simulink model "Estimator_Model_T_variable"  (R2017b)
settings: Solver=FixedStepAuto  StartTime=0.0  StopTime=T  FixedStep=0.01  RelTol=1e-3
values from neighbouring files (symbols this model uses):
  c = 0.02    [mainscript.m]
  Cf = 80000    [Init_for_washout_filter.m]
  Cr = 85000    [Init_for_washout_filter.m]
  L = lf+lr    (= 2.55)    [Init_for_washout_filter.m]
  lf = 0.41*2.55    (= 1.0455)    [Init_for_washout_filter.m]
  lr = 2.55-lf    (= 1.5045)    [Init_for_washout_filter.m]
  m = 3    [mainscript.m]
  mass = 1435-80    (= 1355)    [Init_for_washout_filter.m]
  rollGrad = 5*(pi/180)    (= 0.0872664625997)    [Init_for_washout_filter.m]
  rx = 0.4    [Init_for_washout_filter.m]
  T_w = 1    [mainscript.m]
  Tau = 0.3    [mainscript.m]
settings Model: Creator=gandh  LastModifiedBy=gandh

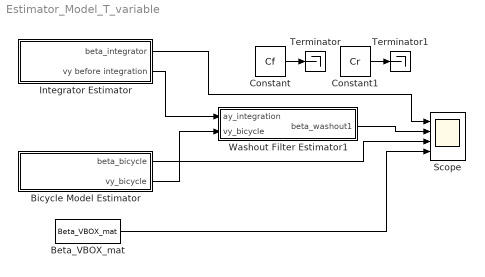
== system Estimator_Model_T_variable ==
  Beta_VBOX_mat : FromWorkspace  VariableName=Beta_VBOX_mat  SampleTime=0
  Bicycle Model Estimator : Subsystem
  Constant : Constant  Value=Cf
  Constant1 : Constant  Value=Cr
  Integrator Estimator : Subsystem
  Scope : Scope  NumInputPorts=4
  Terminator : Terminator
  Terminator1 : Terminator
  Washout Filter Estimator1 : Subsystem
  wires:
  Integrator Estimator/1(beta_integrator) -> Scope/1
  Bicycle Model Estimator/2(vy_bicycle) -> Washout Filter Estimator1/2(vy_bicycle)
  Beta_VBOX_mat/1 -> Scope/4
  Bicycle Model Estimator/1(beta_bicycle) -> Scope/3
  Constant/1 -> Terminator/1
  Constant1/1 -> Terminator1/1
  Integrator Estimator/2(vy before integration) -> Washout Filter Estimator1/1(ay_integration)
  Washout Filter Estimator1/1(beta_washout1) -> Scope/2

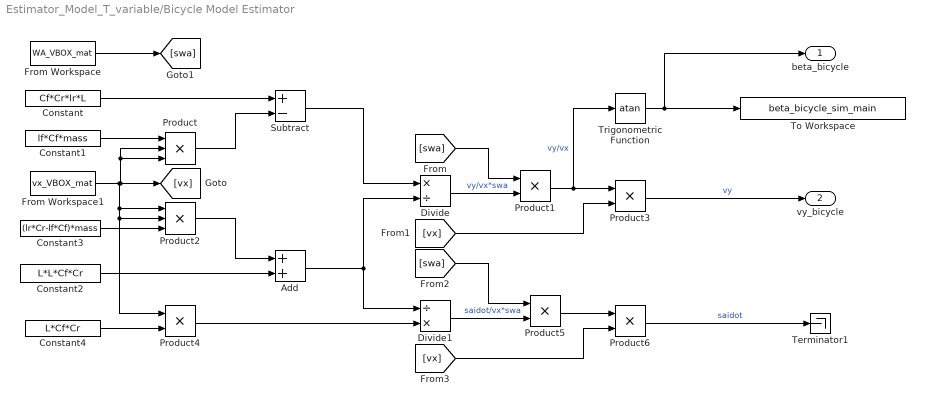
== system Estimator_Model_T_variable/Bicycle Model Estimator ==
  Add : Sum
  Constant : Constant  Value=Cf*Cr*lr*L
  Constant1 : Constant  Value=lf*Cf*mass
  Constant2 : Constant  Value=L*L*Cf*Cr
  Constant3 : Constant  Value=(lr*Cr-lf*Cf)*mass
  Constant4 : Constant  Value=L*Cf*Cr
  Divide : Product  Inputs=*/
  Divide1 : Product  Inputs=/*
  From Workspace : FromWorkspace  VariableName=WA_VBOX_mat  SampleTime=0
  From Workspace1 : FromWorkspace  VariableName=vx_VBOX_mat  SampleTime=0
  Product : Product  Inputs=3
  Product{1,3..6} (5 alike) : Product
  Product2 : Product  Inputs=3
  Subtract : Sum  Inputs=+-
  Terminator1 : Terminator
  To Workspace : ToWorkspace  VariableName=beta_bicycle_sim_main  SaveFormat=Timeseries  SampleTime=-1
  Trigonometric Function : Trigonometry  Operator=atan
  beta_bicycle : Outport
  vy_bicycle : Outport  Port=2
  wires:
  [vx] -> Product3/2
  Constant2/1 -> Add/2
  Product1/1 -> Trigonometric Function/1, Product3/1  "vy/vx"
  Add/1 -> Divide1/1, Divide/2
  Trigonometric Function/1 -> beta_bicycle/1, To Workspace/1
  Constant/1 -> Subtract/1
  Product3/1 -> vy_bicycle/1  "vy"
  Divide1/1 -> Product5/2  "saidot/vx*swa"
  [swa] -> Product1/1
  From Workspace1/1 -> Product2/2, Product4/1, Product2/1, [vx], Product/3, Product/2
  Product6/1 -> Terminator1/1  "saidot"
  Constant1/1 -> Product/1
  Constant4/1 -> Product4/2
  From Workspace/1 -> [swa]
  Divide/1 -> Product1/2  "vy/vx*swa"
  Product/1 -> Subtract/2
  Constant3/1 -> Product2/3
  Product5/1 -> Product6/1
  Product2/1 -> Add/1
  Subtract/1 -> Divide/1
  [vx] -> Product6/2
  [swa] -> Product5/1
  Product4/1 -> Divide1/2

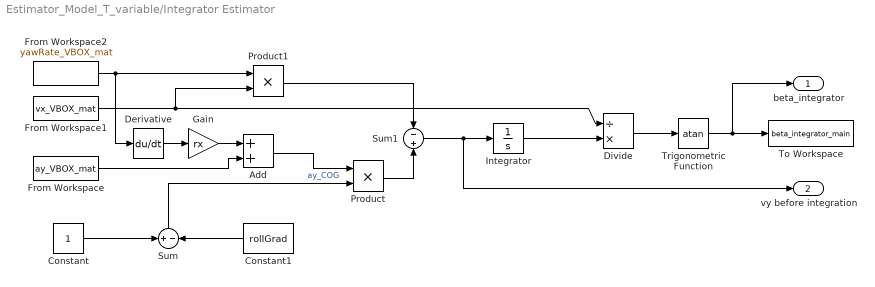
== system Estimator_Model_T_variable/Integrator Estimator ==
  Add : Sum
  Constant : Constant
  Constant1 : Constant  Value=rollGrad
  Derivative : Derivative
  Divide : Product  Inputs=/*
  From Workspace : FromWorkspace  VariableName=ay_VBOX_mat  SampleTime=0
  From Workspace1 : FromWorkspace  VariableName=vx_VBOX_mat  SampleTime=0
  From Workspace2 : FromWorkspace  VariableName=yawRate_VBOX_mat  SampleTime=0
  Gain : Gain  Gain=rx
  Integrator : Integrator
  Product : Product
  Product1 : Product
  Sum : Sum  Inputs=+-
  Sum1 : Sum  Inputs=-+
  To Workspace : ToWorkspace  VariableName=beta_integrator_main  SaveFormat=Timeseries  SampleTime=-1
  Trigonometric Function : Trigonometry  Operator=atan
  beta_integrator : Outport
  vy before integration : Outport  Port=2
  wires:
  Trigonometric Function/1 -> beta_integrator/1, To Workspace/1
  From Workspace1/1 -> Divide/1, Product1/2
  Constant/1 -> Sum/1
  Product/1 -> Sum1/2
  Constant1/1 -> Sum/2
  Product1/1 -> Sum1/1
  Divide/1 -> Trigonometric Function/1
  Sum/1 -> Product/2
  Integrator/1 -> Divide/2
  Add/1 -> Product/1  "ay_COG"
  Derivative/1 -> Gain/1
  From Workspace2/1 -> Derivative/1, Product1/1
  Gain/1 -> Add/1
  From Workspace/1 -> Add/2
  Sum1/1 -> vy before integration/1, Integrator/1

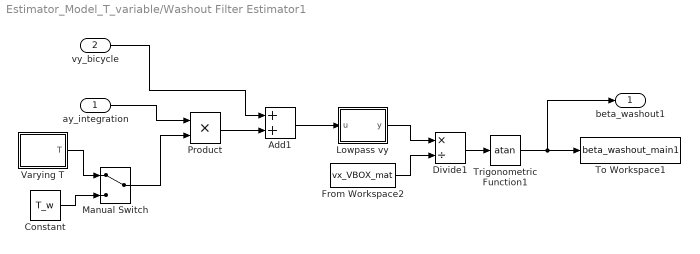
== system Estimator_Model_T_variable/Washout Filter Estimator1 ==
  ay_integration : Inport
  vy_bicycle : Inport  Port=2
  Add1 : Sum
  Constant : Constant  Value=T_w
  Divide1 : Product  Inputs=*/
  From Workspace2 : FromWorkspace  VariableName=vx_VBOX_mat  SampleTime=0
  Lowpass vy : Subsystem
  Manual Switch : ManualSwitch
  Product : Product
  To Workspace1 : ToWorkspace  VariableName=beta_washout_main1  SaveFormat=Timeseries  SampleTime=-1
  Trigonometric Function1 : Trigonometry  Operator=atan
  Varying T : Subsystem
  beta_washout1 : Outport
  wires:
  vy_bicycle/1 -> Add1/1
  ay_integration/1 -> Product/1
  Product/1 -> Add1/2
  Add1/1 -> Lowpass vy/1(u)
  Trigonometric Function1/1 -> To Workspace1/1, beta_washout1/1
  Divide1/1 -> Trigonometric Function1/1
  From Workspace2/1 -> Divide1/2
  Lowpass vy/1(y) -> Divide1/1
  Varying T/1(T) -> Manual Switch/1
  Constant/1 -> Manual Switch/2
  Manual Switch/1 -> Product/2

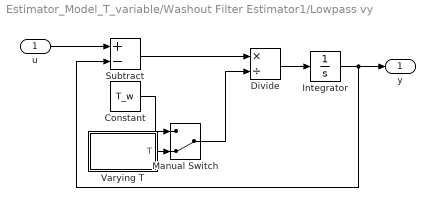
== system Estimator_Model_T_variable/Washout Filter Estimator1/Lowpass vy ==
  u : Inport
  Constant : Constant  Value=T_w
  Divide : Product  Inputs=*/
  Integrator : Integrator
  Manual Switch : ManualSwitch  CurrentSetting=0
  Subtract : Sum  Inputs=+-
  Varying T : Subsystem
  y : Outport
  wires:
  Divide/1 -> Integrator/1
  u/1 -> Subtract/1
  Subtract/1 -> Divide/1
  Integrator/1 -> Subtract/2, y/1
  Varying T/1(T) -> Manual Switch/2
  Manual Switch/1 -> Divide/2
  Constant/1 -> Manual Switch/1

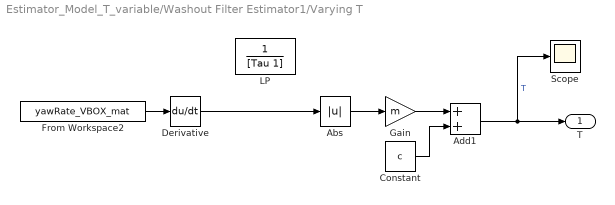
== system Estimator_Model_T_variable/Washout Filter Estimator1/Varying T ==
  Abs : Abs
  Add1 : Sum
  Constant : Constant  Value=c
  Derivative : Derivative
  From Workspace2 : FromWorkspace  VariableName=yawRate_VBOX_mat  SampleTime=0
  Gain : Gain  Gain=m
  LP : TransferFcn  Denominator=[Tau 1]
  Scope : Scope
  T : Outport
  wires:
  Gain/1 -> Add1/1
  Add1/1 -> Scope/1, T/1  "T"
  Abs/1 -> Gain/1
  From Workspace2/1 -> Derivative/1
  Constant/1 -> Add1/2
  Derivative/1 -> Abs/1

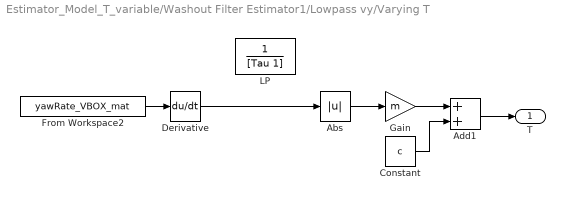
== system Estimator_Model_T_variable/Washout Filter Estimator1/Lowpass vy/Varying T ==
  Abs : Abs
  Add1 : Sum
  Constant : Constant  Value=c
  Derivative : Derivative
  From Workspace2 : FromWorkspace  VariableName=yawRate_VBOX_mat  SampleTime=0
  Gain : Gain  Gain=m
  LP : TransferFcn  Denominator=[Tau 1]
  T : Outport
  wires:
  Gain/1 -> Add1/1
  Add1/1 -> T/1
  Abs/1 -> Gain/1
  From Workspace2/1 -> Derivative/1
  Constant/1 -> Add1/2
  Derivative/1 -> Abs/1
